simulink model "CAN_Model_v5"  (R2018b)
settings: Solver=VariableStepAuto  StartTime=0.0  StopTime=SimTime  RelTol=1e-3
InitFcn:
  | run('CAN_ModelMat.m')
values from neighbouring files (symbols this model uses):
  ID = [1,0,0,0,0,1,1,0,0,1,0]    [CAN_ModelMat.m]    (also in CAN_ModelMatv2.m = [1,1,1,1,1,0,0,1,1,1,1]; stuff.m = [ID(1:i) 0 ID(i+1:end)])
  NodesID = [ 0,0,1,1,0,1,1,0,0,1,1 ... (first row only)    [CAN_ModelMat.m]    (also in CAN_ModelMatv2.m)
  RandPayload = randi([0,1],1, 64)    [CAN_ModelMat.m]
  RTS_Inc = round(SimTime / CLK / NumOfFrames)    [CAN_ModelMat.m]    (also in CAN_ModelMatv2.m)
  time = NodeTiming / CLK    (= 5000)    [CAN_ModelMat.m]    (also in CAN_ModelMatv2.m)
libraries: simulink_extras x1
settings Model: Creator=Emiliano  LastModifiedBy=MAX_1

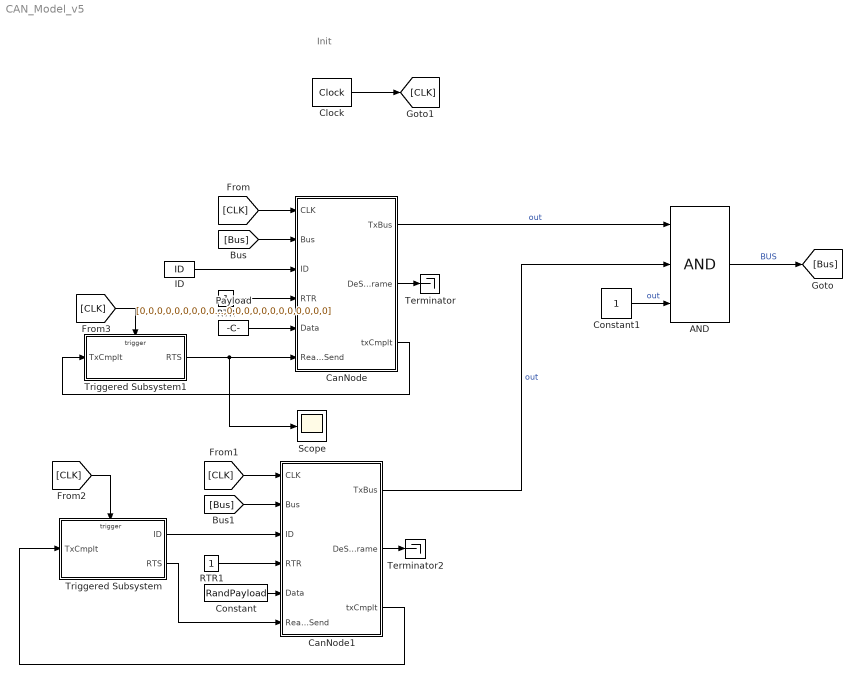
== system CAN_Model_v5 ==
  note: Init
  AND : Logic  Inputs=3  IconShape=distinctive  AllPortsSameDT=off  OutDataTypeStr=boolean
  CanNode : Subsystem
  CanNode1 : Subsystem
  Clock : simulink_extras/Flip Flops/Clock  period=CLK
  Constant : Constant  Value=RandPayload
  Constant1 : Constant
  ID : Constant  Value=ID
  "Payload " : Constant  Value=[0,0,0,0,0,0,0,0,0,0,0,0,0,0,0,0,0,0,0,0,0,0,0,0,0,0,0,0,0,0,0,0,0,0,0,0,0,0,0,0,0,0,0,0,0,0,0,0,0,0,0,0,0,0,0,0,0,0,0,0,0,0,0,0]
  RTR : Constant
  RTR1 : Constant
  Scope : Scope
  Terminator : Terminator
  Terminator2 : Terminator
  Triggered Subsystem : Subsystem  TreatAsAtomicUnit=on
  Triggered Subsystem1 : Subsystem  TreatAsAtomicUnit=on
  wires:
  CanNode/1("TxBus ") -> AND/1  "out"
  [Bus] -> CanNode/2(Bus)
  Triggered Subsystem1/1(RTS) -> Scope/1, CanNode/6("ReadyToSend ")
  ID/1 -> CanNode/3(ID)
  "Payload "/1 -> CanNode/5(Data)
  RTR/1 -> CanNode/4(RTR)
  Constant1/1 -> AND/3  "out"
  AND/1 -> [Bus]  "BUS"
  Clock/1 -> [CLK]
  [CLK] -> CanNode/1(CLK)
  CanNode/2(DeStuffedFrame) -> Terminator/1
  Triggered Subsystem/2(RTS) -> CanNode1/6("ReadyToSend ")
  [CLK] -> CanNode1/1(CLK)
  [Bus] -> CanNode1/2(Bus)
  CanNode1/1("TxBus ") -> AND/2  "out"
  CanNode1/3(txCmplt) -> Triggered Subsystem/1(TxCmplt)
  RTR1/1 -> CanNode1/4(RTR)
  CanNode1/2(DeStuffedFrame) -> Terminator2/1
  [CLK] -> Triggered Subsystem/Trigger
  Triggered Subsystem/1(ID) -> CanNode1/3(ID)
  [CLK] -> Triggered Subsystem1/Trigger
  CanNode/3(txCmplt) -> Triggered Subsystem1/1(TxCmplt)
  Constant/1 -> CanNode1/5(Data)

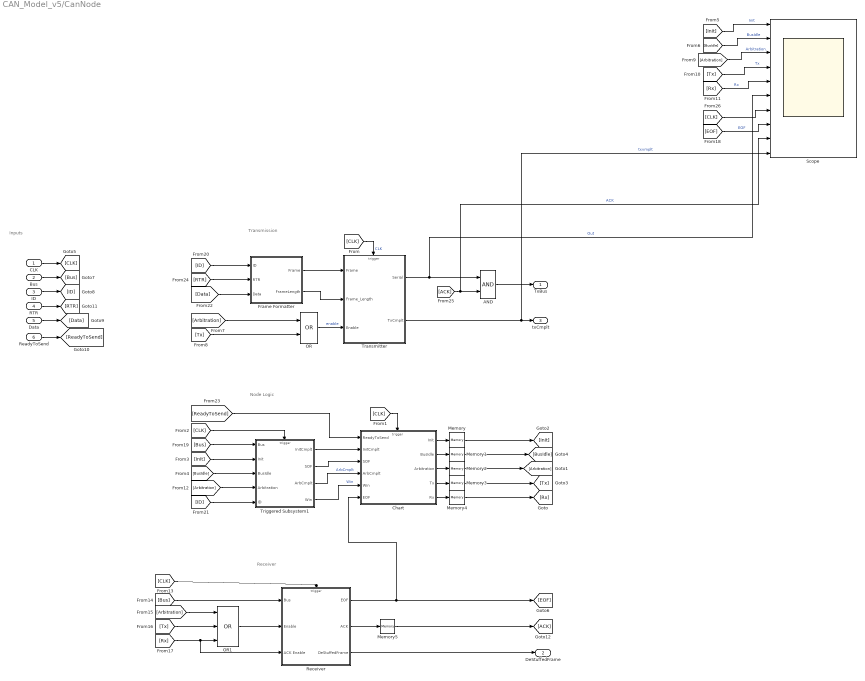
== system CAN_Model_v5/CanNode ==
  note: Transmission
  note: Node Logic
  note: Receiver
  note: Inputs
  CLK : Inport
  Bus : Inport  Port=2
  ID : Inport  Port=3
  RTR : Inport  Port=4
  Data : Inport  Port=5
  "ReadyToSend " : Inport  Port=6
  AND : Logic  IconShape=distinctive  AllPortsSameDT=off  OutDataTypeStr=boolean
  Chart : Stateflow chart  TreatAsAtomicUnit=on
  Frame Formatter : Subsystem
  Memory{,1..5} (6 alike) : Memory
  OR : Logic  Operator=OR  IconShape=distinctive  AllPortsSameDT=off  OutDataTypeStr=boolean
  OR1 : Logic  Operator=OR  Inputs=3  IconShape=distinctive  AllPortsSameDT=off  OutDataTypeStr=boolean
  Receiver : Subsystem  TreatAsAtomicUnit=on
  Scope : Scope  NumInputPorts=10
  Transmitter : Subsystem  TreatAsAtomicUnit=on
  Triggered Subsystem1 : Subsystem  TreatAsAtomicUnit=on
  "TxBus " : Outport
  DeStuffedFrame : Outport  Port=2
  txCmplt : Outport  Port=3
  wires:
  [CLK] -> Chart/Trigger
  [Arbitration] -> OR/1
  [Tx] -> OR/2
  OR/1 -> Transmitter/3(Enable)  "enable"
  Chart/5(" Rx") -> Memory4/1
  Chart/3(" Arbitration") -> Memory2/1
  Chart/1(" Init") -> Memory/1
  Chart/4(" Tx") -> Memory3/1
  Chart/2(" BusIdle") -> Memory1/1
  CLK/1 -> [CLK]
  [CLK] -> Transmitter/Trigger  "CLK"
  [CLK] -> Triggered Subsystem1/Trigger
  [Init] -> Triggered Subsystem1/2(Init)
  [BusIdle] -> Triggered Subsystem1/3(BusIdle)
  Triggered Subsystem1/2(SOF) -> Chart/3(SOF)
  Triggered Subsystem1/3("ArbCmplt ") -> Chart/4(ArbCmplt)  "ArbCmplt"
  [Init] -> Scope/1  "Init"
  [BusIdle] -> Scope/2  "BusIdle"
  [Arbitration] -> Scope/3  "Arbitration"
  [Tx] -> Scope/4  "Tx"
  [Rx] -> Scope/5  "Rx"
  Memory/1 -> [Init]
  Memory1/1 -> [BusIdle]
  Memory2/1 -> [Arbitration]
  Memory3/1 -> [Tx]
  Memory4/1 -> [Rx]
  Transmitter/1(Serial) -> Scope/6, AND/1  "Out"
  [Arbitration] -> Triggered Subsystem1/4(Arbitration)
  [CLK] -> Receiver/Trigger
  [Bus] -> Receiver/1(Bus)
  [Arbitration] -> OR1/1
  [Tx] -> OR1/2
  Receiver/1(EOF) -> Chart/6(EOF), [EOF]
  [EOF] -> Scope/8  "EOF"
  Bus/1 -> [Bus]
  [Bus] -> Triggered Subsystem1/1(Bus)
  Frame Formatter/1(Frame) -> Transmitter/1("Frame ")
  Frame Formatter/2("FrameLength ") -> Transmitter/2(Frame_Length)
  ID/1 -> [ID]
  [ID] -> Frame Formatter/1(ID)
  [ID] -> Triggered Subsystem1/5(ID)
  Data/1 -> [Data]
  "ReadyToSend "/1 -> [ReadyToSend]
  [ReadyToSend] -> Chart/1(ReadyToSend)
  [Data] -> Frame Formatter/3(Data)
  RTR/1 -> [RTR]
  [RTR] -> Frame Formatter/2(RTR)
  Receiver/2(ACK) -> Memory5/1
  Triggered Subsystem1/4(Win) -> Chart/5(Win)  "Win"
  Memory5/1 -> [ACK]
  AND/1 -> "TxBus "/1
  [ACK] -> Scope/9, AND/2  "ACK"
  Triggered Subsystem1/1(InitCmplt) -> Chart/2(InitCmplt)
  [CLK] -> Scope/7
  Receiver/3(DeStuffedFrame) -> DeStuffedFrame/1
  OR1/1 -> Receiver/2(Enable)
  [Rx] -> Receiver/3(ACK Enable), OR1/3
  Transmitter/2(TxCmplt) -> Scope/10, txCmplt/1  "txvmplt"

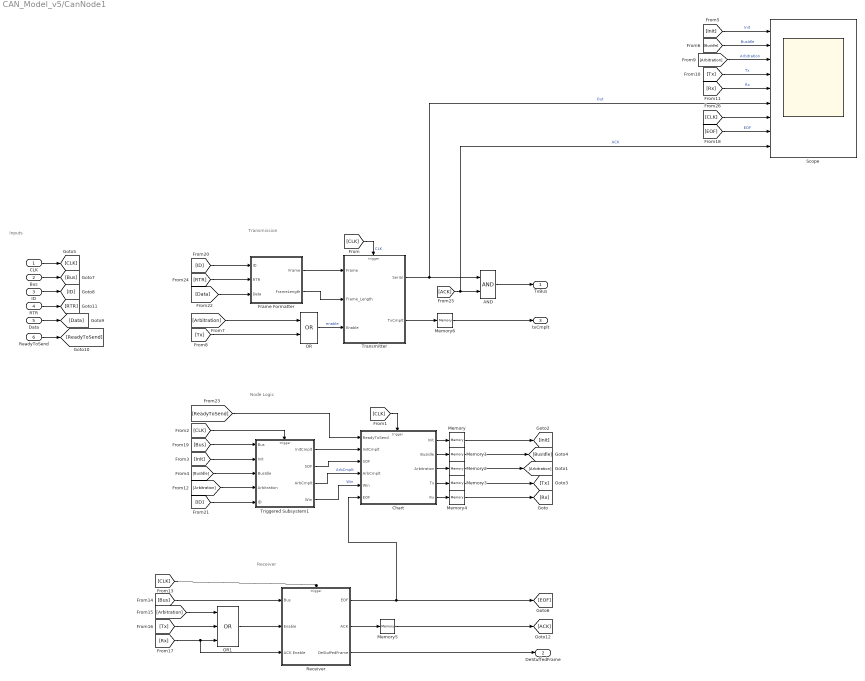
== system CAN_Model_v5/CanNode1 ==
  note: Transmission
  note: Node Logic
  note: Receiver
  note: Inputs
  CLK : Inport
  Bus : Inport  Port=2
  ID : Inport  Port=3
  RTR : Inport  Port=4
  Data : Inport  Port=5
  "ReadyToSend " : Inport  Port=6
  AND : Logic  IconShape=distinctive  AllPortsSameDT=off  OutDataTypeStr=boolean
  Chart : Stateflow chart  TreatAsAtomicUnit=on
  Frame Formatter : Subsystem
  Memory{,1..6} (7 alike) : Memory
  OR : Logic  Operator=OR  IconShape=distinctive  AllPortsSameDT=off  OutDataTypeStr=boolean
  OR1 : Logic  Operator=OR  Inputs=3  IconShape=distinctive  AllPortsSameDT=off  OutDataTypeStr=boolean
  Receiver : Subsystem  TreatAsAtomicUnit=on
  Scope : Scope  NumInputPorts=9
  Transmitter : Subsystem  TreatAsAtomicUnit=on
  Triggered Subsystem1 : Subsystem  TreatAsAtomicUnit=on
  "TxBus " : Outport
  DeStuffedFrame : Outport  Port=2
  txCmplt : Outport  Port=3
  wires:
  [CLK] -> Chart/Trigger
  [Arbitration] -> OR/1
  [Tx] -> OR/2
  OR/1 -> Transmitter/3(Enable)  "enable"
  Chart/5(" Rx") -> Memory4/1
  Chart/3(" Arbitration") -> Memory2/1
  Chart/1(" Init") -> Memory/1
  Chart/4(" Tx") -> Memory3/1
  Chart/2(" BusIdle") -> Memory1/1
  CLK/1 -> [CLK]
  [CLK] -> Transmitter/Trigger  "CLK"
  [CLK] -> Triggered Subsystem1/Trigger
  [Init] -> Triggered Subsystem1/2(Init)
  [BusIdle] -> Triggered Subsystem1/3(BusIdle)
  Triggered Subsystem1/2(SOF) -> Chart/3(SOF)
  Triggered Subsystem1/3("ArbCmplt ") -> Chart/4(ArbCmplt)  "ArbCmplt"
  [Init] -> Scope/1  "Init"
  [BusIdle] -> Scope/2  "BusIdle"
  [Arbitration] -> Scope/3  "Arbitration"
  [Tx] -> Scope/4  "Tx"
  [Rx] -> Scope/5  "Rx"
  Memory/1 -> [Init]
  Memory1/1 -> [BusIdle]
  Memory2/1 -> [Arbitration]
  Memory3/1 -> [Tx]
  Memory4/1 -> [Rx]
  Transmitter/1(Serial) -> Scope/6, AND/1  "Out"
  [Arbitration] -> Triggered Subsystem1/4(Arbitration)
  [CLK] -> Receiver/Trigger
  [Bus] -> Receiver/1(Bus)
  [Arbitration] -> OR1/1
  [Tx] -> OR1/2
  Receiver/1(EOF) -> Chart/6(EOF), [EOF]
  [EOF] -> Scope/8  "EOF"
  Bus/1 -> [Bus]
  [Bus] -> Triggered Subsystem1/1(Bus)
  Frame Formatter/1(Frame) -> Transmitter/1("Frame ")
  Frame Formatter/2("FrameLength ") -> Transmitter/2(Frame_Length)
  ID/1 -> [ID]
  [ID] -> Frame Formatter/1(ID)
  [ID] -> Triggered Subsystem1/5(ID)
  Data/1 -> [Data]
  "ReadyToSend "/1 -> [ReadyToSend]
  [ReadyToSend] -> Chart/1(ReadyToSend)
  [Data] -> Frame Formatter/3(Data)
  RTR/1 -> [RTR]
  [RTR] -> Frame Formatter/2(RTR)
  Receiver/2(ACK) -> Memory5/1
  Triggered Subsystem1/4(Win) -> Chart/5(Win)  "Win"
  Memory5/1 -> [ACK]
  AND/1 -> "TxBus "/1
  [ACK] -> Scope/9, AND/2  "ACK"
  Triggered Subsystem1/1(InitCmplt) -> Chart/2(InitCmplt)
  [CLK] -> Scope/7
  Receiver/3(DeStuffedFrame) -> DeStuffedFrame/1
  OR1/1 -> Receiver/2(Enable)
  [Rx] -> Receiver/3(ACK Enable), OR1/3
  Transmitter/2(TxCmplt) -> Memory6/1
  Memory6/1 -> txCmplt/1

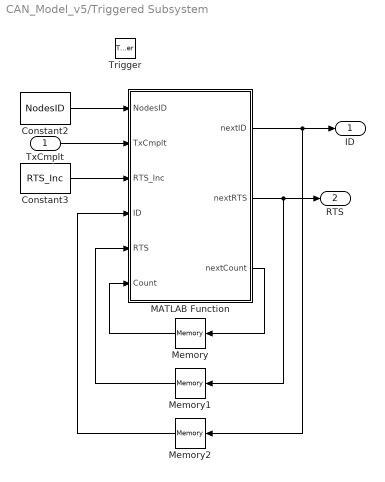
== system CAN_Model_v5/Triggered Subsystem ==
  TxCmplt : Inport
  Trigger : TriggerPort  VariantControl=Variant
  Constant2 : Constant  Value=NodesID
  Constant3 : Constant  Value=RTS_Inc
  MATLAB Function : MATLAB Function  TreatAsAtomicUnit=on
  Memory : Memory  InheritSampleTime=on
  Memory1 : Memory  InheritSampleTime=on
  Memory2 : Memory  InitialCondition=NodesID(1,:)  InheritSampleTime=on
  ID : Outport
  RTS : Outport  Port=2
  wires:
  Constant2/1 -> MATLAB Function/1(NodesID)
  MATLAB Function/3(nextCount) -> Memory/1
  Memory/1 -> MATLAB Function/6(Count)
  MATLAB Function/2(nextRTS) -> RTS/1, Memory1/1
  Memory1/1 -> MATLAB Function/5(RTS)
  MATLAB Function/1(nextID) -> ID/1, Memory2/1
  Memory2/1 -> MATLAB Function/4(ID)
  Constant3/1 -> MATLAB Function/3(RTS_Inc)
  TxCmplt/1 -> MATLAB Function/2(TxCmplt)

== system CAN_Model_v5/Triggered Subsystem1 ==
  TxCmplt : Inport
  Trigger : TriggerPort  VariantControl=Variant
  Constant : Constant  Value=time
  MATLAB Function : MATLAB Function  TreatAsAtomicUnit=on
  Memory : Memory  InheritSampleTime=on
  Memory1 : Memory  InheritSampleTime=on
  RTS : Outport
  wires:
  MATLAB Function/1(nextRTS) -> Memory1/1, RTS/1
  Constant/1 -> MATLAB Function/1(Timer)
  TxCmplt/1 -> MATLAB Function/2(TxCmplt)
  MATLAB Function/2(nextCount) -> Memory/1
  Memory/1 -> MATLAB Function/4(Count)
  Memory1/1 -> MATLAB Function/3(RTS)

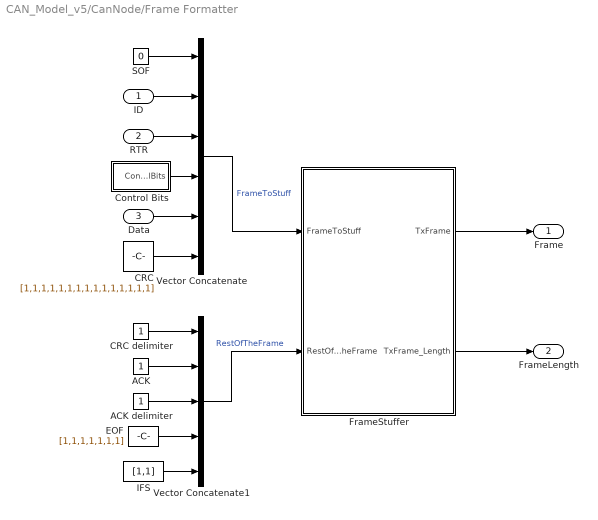
== system CAN_Model_v5/CanNode/Frame Formatter ==
  ID : Inport
  RTR : Inport  Port=2
  Data : Inport  Port=3
  ACK : Constant
  ACK delimiter : Constant
  CRC : Constant  Value=[1,1,1,1,1,1,1,1,1,1,1,1,1,1,1]
  CRC delimiter : Constant  VectorParams1D=off
  Control Bits : Subsystem
  EOF : Constant  Value=[1,1,1,1,1,1,1]
  FrameStuffer : Subsystem
  IFS : Constant  Value=[1,1]
  SOF : Constant  Value=0
  Vector Concatenate : Concatenate  NumInputs=6
  Vector Concatenate1 : Concatenate  NumInputs=5
  Frame : Outport
  "FrameLength " : Outport  Port=2
  wires:
  ID/1 -> Vector Concatenate/2
  RTR/1 -> Vector Concatenate/3
  Vector Concatenate/1 -> FrameStuffer/1(FrameToStuff)  "FrameToStuff"
  FrameStuffer/1(TxFrame) -> Frame/1
  FrameStuffer/2(TxFrame_Length) -> "FrameLength "/1
  SOF/1 -> Vector Concatenate/1
  Control Bits/1(ControlBits) -> Vector Concatenate/4
  Data/1 -> Vector Concatenate/5
  CRC/1 -> Vector Concatenate/6
  CRC delimiter/1 -> Vector Concatenate1/1
  ACK/1 -> Vector Concatenate1/2
  ACK delimiter/1 -> Vector Concatenate1/3
  EOF/1 -> Vector Concatenate1/4
  IFS/1 -> Vector Concatenate1/5
  Vector Concatenate1/1 -> FrameStuffer/2(RestOfTheFrame)  "RestOfTheFrame"

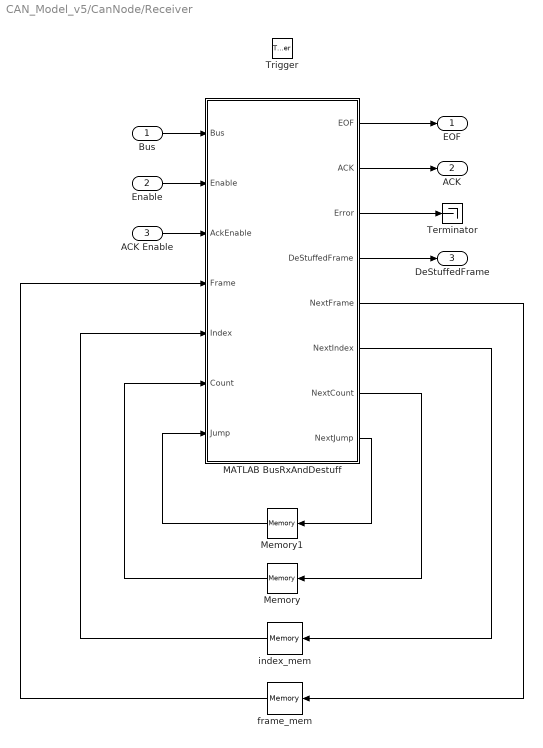
== system CAN_Model_v5/CanNode/Receiver ==
  Bus : Inport
  Enable : Inport  Port=2
  ACK Enable : Inport  Port=3
  Trigger : TriggerPort  VariantControl=Variant
  MATLAB BusRxAndDestuff : MATLAB Function  TreatAsAtomicUnit=on
  Memory : Memory  InheritSampleTime=on
  Memory1 : Memory  InheritSampleTime=on
  Terminator : Terminator
  frame_mem : Memory  InitialCondition=[0,0,0,0,0,0,0,0,0,0,0,0,0,0,0,0,0,0,0,0,0,0,0,0,0,0,0,0,0,0,0,0,0,0,0,0,0,0,0,0,0,0,0,0,0,0,0,0,0,0,0,0,0,0,0,0,0,0,0,0,0,0,0,0,0,0,0,0,0,0,0,0,0,0,0,0,0,0,0,0,0,0,0,0,0,0,0,0,0,0,0,0,0,0,0,0,0,0,0,0,0,0,0,0,0,0,0,0,0,0]  InheritSampleTime=on
  index_mem : Memory  InitialCondition=1  InheritSampleTime=on
  EOF : Outport
  ACK : Outport  Port=2
  DeStuffedFrame : Outport  Port=3
  wires:
  Enable/1 -> MATLAB BusRxAndDestuff/2(Enable)
  Bus/1 -> MATLAB BusRxAndDestuff/1(Bus)
  MATLAB BusRxAndDestuff/6(NextIndex) -> index_mem/1
  frame_mem/1 -> MATLAB BusRxAndDestuff/4(Frame)
  MATLAB BusRxAndDestuff/1(EOF) -> EOF/1
  MATLAB BusRxAndDestuff/5(NextFrame) -> frame_mem/1
  index_mem/1 -> MATLAB BusRxAndDestuff/5(Index)
  MATLAB BusRxAndDestuff/3(Error) -> Terminator/1
  MATLAB BusRxAndDestuff/7(NextCount) -> Memory/1
  Memory/1 -> MATLAB BusRxAndDestuff/6(Count)
  MATLAB BusRxAndDestuff/8(NextJump) -> Memory1/1
  Memory1/1 -> MATLAB BusRxAndDestuff/7(Jump)
  MATLAB BusRxAndDestuff/4(DeStuffedFrame) -> DeStuffedFrame/1
  MATLAB BusRxAndDestuff/2(ACK) -> ACK/1
  ACK Enable/1 -> MATLAB BusRxAndDestuff/3(AckEnable)

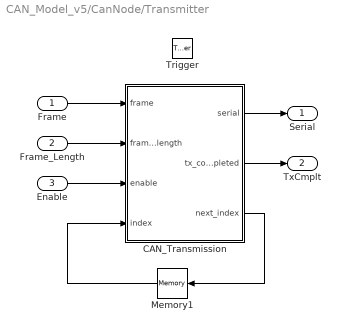
== system CAN_Model_v5/CanNode/Transmitter ==
  "Frame " : Inport
  Frame_Length : Inport  Port=2
  Enable : Inport  Port=3
  Trigger : TriggerPort  VariantControl=Variant
  CAN_Transmission : MATLAB Function  TreatAsAtomicUnit=on
  Memory1 : Memory  InitialCondition=1  InheritSampleTime=on
  Serial : Outport
  TxCmplt : Outport  Port=2
  wires:
  Memory1/1 -> CAN_Transmission/4(index)
  CAN_Transmission/1(serial) -> Serial/1
  CAN_Transmission/3(next_index) -> Memory1/1
  CAN_Transmission/2(tx_completed) -> TxCmplt/1
  Enable/1 -> CAN_Transmission/3(enable)
  "Frame "/1 -> CAN_Transmission/1(frame)
  Frame_Length/1 -> CAN_Transmission/2(frame_length)

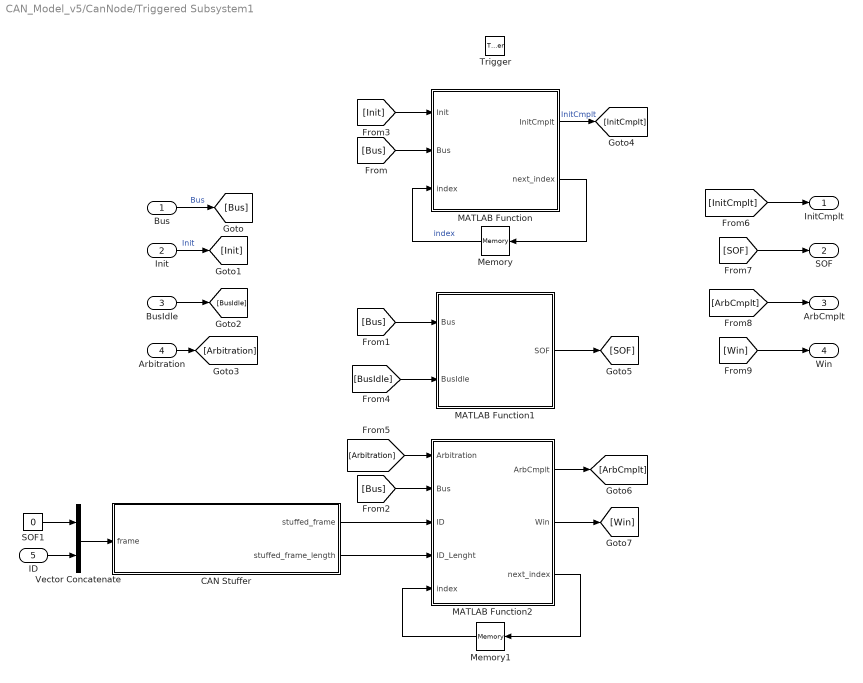
== system CAN_Model_v5/CanNode/Triggered Subsystem1 ==
  Bus : Inport
  Init : Inport  Port=2
  BusIdle : Inport  Port=3
  Arbitration : Inport  Port=4
  ID : Inport  Port=5
  Trigger : TriggerPort  VariantControl=Variant
  CAN Stuffer : MATLAB Function  TreatAsAtomicUnit=on
  MATLAB Function : MATLAB Function  TreatAsAtomicUnit=on
  MATLAB Function1 : MATLAB Function  TreatAsAtomicUnit=on
  MATLAB Function2 : MATLAB Function  TreatAsAtomicUnit=on
  Memory : Memory  InheritSampleTime=on
  Memory1 : Memory  InitialCondition=1  InheritSampleTime=on
  SOF1 : Constant  Value=0
  Vector Concatenate : Concatenate
  InitCmplt : Outport
  SOF : Outport  Port=2
  "ArbCmplt " : Outport  Port=3
  Win : Outport  Port=4
  wires:
  MATLAB Function/2(next_index) -> Memory/1
  Memory/1 -> MATLAB Function/3(index)  "index"
  Bus/1 -> [Bus]  "Bus"
  [Bus] -> MATLAB Function/2(Bus)
  [Bus] -> MATLAB Function1/1(Bus)
  [Bus] -> MATLAB Function2/2(Bus)
  MATLAB Function2/3(next_index) -> Memory1/1
  Memory1/1 -> MATLAB Function2/5(index)
  CAN Stuffer/1(stuffed_frame) -> MATLAB Function2/3(ID)
  CAN Stuffer/2(stuffed_frame_length) -> MATLAB Function2/4(ID_Lenght)
  SOF1/1 -> Vector Concatenate/1
  ID/1 -> Vector Concatenate/2
  Vector Concatenate/1 -> CAN Stuffer/1(frame)
  Init/1 -> [Init]  "Init"
  [Init] -> MATLAB Function/1(Init)
  BusIdle/1 -> [BusIdle]
  [BusIdle] -> MATLAB Function1/2(BusIdle)
  Arbitration/1 -> [Arbitration]
  [Arbitration] -> MATLAB Function2/1(Arbitration)
  MATLAB Function/1(InitCmplt) -> [InitCmplt]  "InitCmplt"
  [InitCmplt] -> InitCmplt/1
  MATLAB Function1/1(SOF) -> [SOF]
  [SOF] -> SOF/1
  MATLAB Function2/1(ArbCmplt) -> [ArbCmplt]
  [ArbCmplt] -> "ArbCmplt "/1
  [Win] -> Win/1
  MATLAB Function2/2(Win) -> [Win]

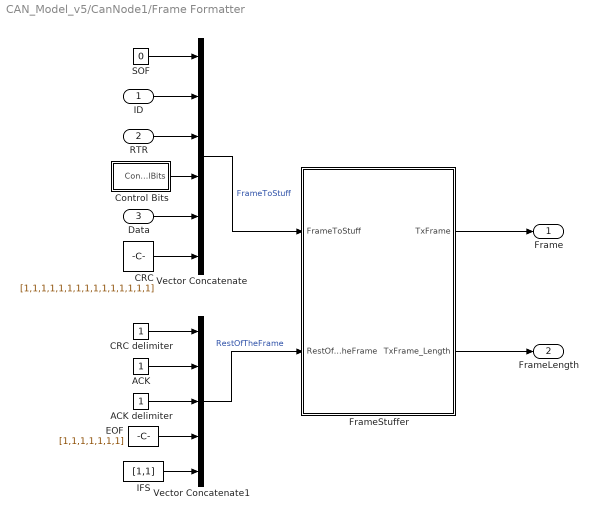
== system CAN_Model_v5/CanNode1/Frame Formatter ==
  ID : Inport
  RTR : Inport  Port=2
  Data : Inport  Port=3
  ACK : Constant
  ACK delimiter : Constant
  CRC : Constant  Value=[1,1,1,1,1,1,1,1,1,1,1,1,1,1,1]
  CRC delimiter : Constant  VectorParams1D=off
  Control Bits : Subsystem
  EOF : Constant  Value=[1,1,1,1,1,1,1]
  FrameStuffer : Subsystem
  IFS : Constant  Value=[1,1]
  SOF : Constant  Value=0
  Vector Concatenate : Concatenate  NumInputs=6
  Vector Concatenate1 : Concatenate  NumInputs=5
  Frame : Outport
  "FrameLength " : Outport  Port=2
  wires:
  ID/1 -> Vector Concatenate/2
  RTR/1 -> Vector Concatenate/3
  Vector Concatenate/1 -> FrameStuffer/1(FrameToStuff)  "FrameToStuff"
  FrameStuffer/1(TxFrame) -> Frame/1
  FrameStuffer/2(TxFrame_Length) -> "FrameLength "/1
  SOF/1 -> Vector Concatenate/1
  Control Bits/1(ControlBits) -> Vector Concatenate/4
  Data/1 -> Vector Concatenate/5
  CRC/1 -> Vector Concatenate/6
  CRC delimiter/1 -> Vector Concatenate1/1
  ACK/1 -> Vector Concatenate1/2
  ACK delimiter/1 -> Vector Concatenate1/3
  EOF/1 -> Vector Concatenate1/4
  IFS/1 -> Vector Concatenate1/5
  Vector Concatenate1/1 -> FrameStuffer/2(RestOfTheFrame)  "RestOfTheFrame"

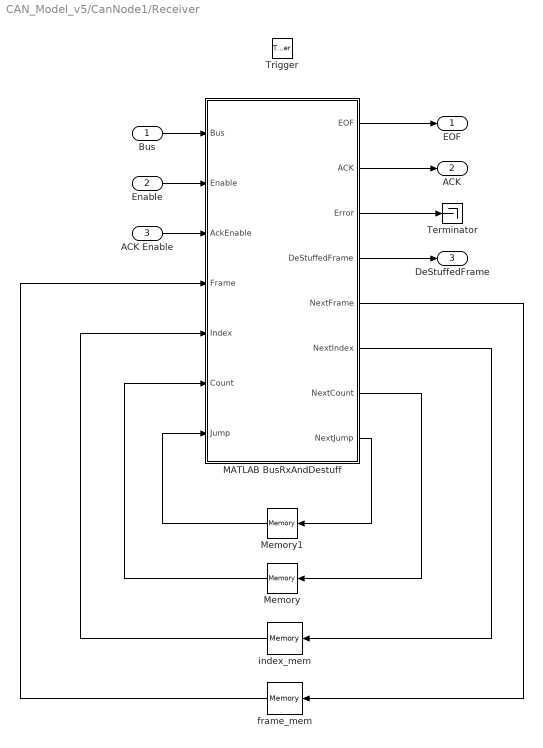
== system CAN_Model_v5/CanNode1/Receiver ==
  Bus : Inport
  Enable : Inport  Port=2
  ACK Enable : Inport  Port=3
  Trigger : TriggerPort  VariantControl=Variant
  MATLAB BusRxAndDestuff : MATLAB Function  TreatAsAtomicUnit=on
  Memory : Memory  InheritSampleTime=on
  Memory1 : Memory  InheritSampleTime=on
  Terminator : Terminator
  frame_mem : Memory  InitialCondition=[0,0,0,0,0,0,0,0,0,0,0,0,0,0,0,0,0,0,0,0,0,0,0,0,0,0,0,0,0,0,0,0,0,0,0,0,0,0,0,0,0,0,0,0,0,0,0,0,0,0,0,0,0,0,0,0,0,0,0,0,0,0,0,0,0,0,0,0,0,0,0,0,0,0,0,0,0,0,0,0,0,0,0,0,0,0,0,0,0,0,0,0,0,0,0,0,0,0,0,0,0,0,0,0,0,0,0,0,0,0]  InheritSampleTime=on
  index_mem : Memory  InitialCondition=1  InheritSampleTime=on
  EOF : Outport
  ACK : Outport  Port=2
  DeStuffedFrame : Outport  Port=3
  wires:
  Enable/1 -> MATLAB BusRxAndDestuff/2(Enable)
  Bus/1 -> MATLAB BusRxAndDestuff/1(Bus)
  MATLAB BusRxAndDestuff/6(NextIndex) -> index_mem/1
  frame_mem/1 -> MATLAB BusRxAndDestuff/4(Frame)
  MATLAB BusRxAndDestuff/1(EOF) -> EOF/1
  MATLAB BusRxAndDestuff/5(NextFrame) -> frame_mem/1
  index_mem/1 -> MATLAB BusRxAndDestuff/5(Index)
  MATLAB BusRxAndDestuff/3(Error) -> Terminator/1
  MATLAB BusRxAndDestuff/7(NextCount) -> Memory/1
  Memory/1 -> MATLAB BusRxAndDestuff/6(Count)
  MATLAB BusRxAndDestuff/8(NextJump) -> Memory1/1
  Memory1/1 -> MATLAB BusRxAndDestuff/7(Jump)
  MATLAB BusRxAndDestuff/4(DeStuffedFrame) -> DeStuffedFrame/1
  MATLAB BusRxAndDestuff/2(ACK) -> ACK/1
  ACK Enable/1 -> MATLAB BusRxAndDestuff/3(AckEnable)

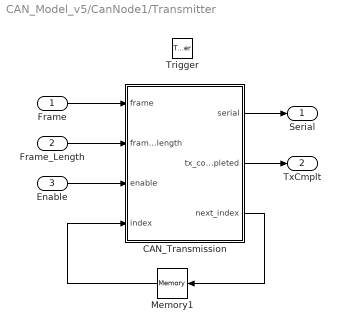
== system CAN_Model_v5/CanNode1/Transmitter ==
  "Frame " : Inport
  Frame_Length : Inport  Port=2
  Enable : Inport  Port=3
  Trigger : TriggerPort  VariantControl=Variant
  CAN_Transmission : MATLAB Function  TreatAsAtomicUnit=on
  Memory1 : Memory  InitialCondition=1  InheritSampleTime=on
  Serial : Outport
  TxCmplt : Outport  Port=2
  wires:
  Memory1/1 -> CAN_Transmission/4(index)
  CAN_Transmission/1(serial) -> Serial/1
  CAN_Transmission/3(next_index) -> Memory1/1
  CAN_Transmission/2(tx_completed) -> TxCmplt/1
  Enable/1 -> CAN_Transmission/3(enable)
  "Frame "/1 -> CAN_Transmission/1(frame)
  Frame_Length/1 -> CAN_Transmission/2(frame_length)

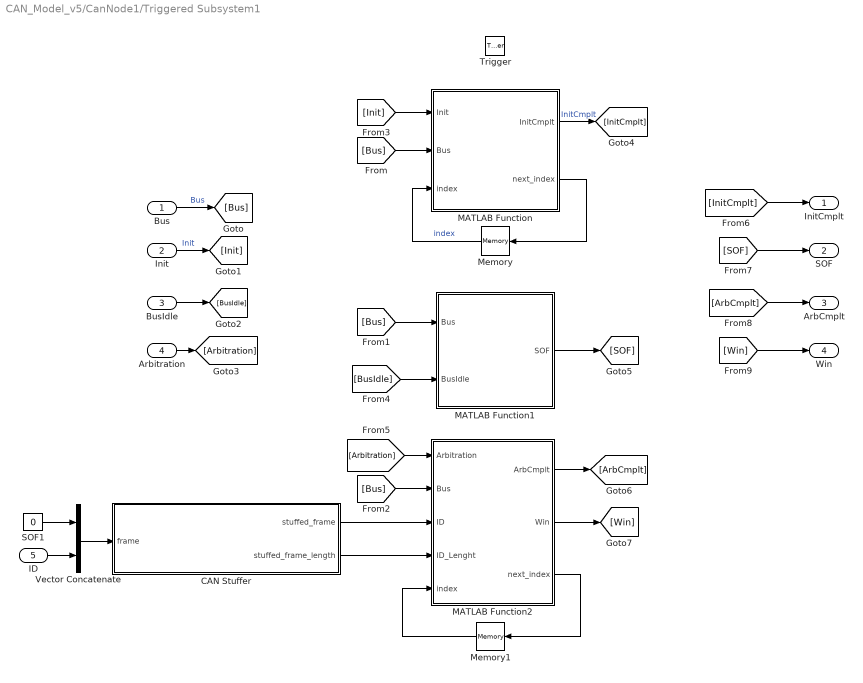
== system CAN_Model_v5/CanNode1/Triggered Subsystem1 ==
  Bus : Inport
  Init : Inport  Port=2
  BusIdle : Inport  Port=3
  Arbitration : Inport  Port=4
  ID : Inport  Port=5
  Trigger : TriggerPort  VariantControl=Variant
  CAN Stuffer : MATLAB Function  TreatAsAtomicUnit=on
  MATLAB Function : MATLAB Function  TreatAsAtomicUnit=on
  MATLAB Function1 : MATLAB Function  TreatAsAtomicUnit=on
  MATLAB Function2 : MATLAB Function  TreatAsAtomicUnit=on
  Memory : Memory  InheritSampleTime=on
  Memory1 : Memory  InitialCondition=1  InheritSampleTime=on
  SOF1 : Constant  Value=0
  Vector Concatenate : Concatenate
  InitCmplt : Outport
  SOF : Outport  Port=2
  "ArbCmplt " : Outport  Port=3
  Win : Outport  Port=4
  wires:
  MATLAB Function/2(next_index) -> Memory/1
  Memory/1 -> MATLAB Function/3(index)  "index"
  Bus/1 -> [Bus]  "Bus"
  [Bus] -> MATLAB Function/2(Bus)
  [Bus] -> MATLAB Function1/1(Bus)
  [Bus] -> MATLAB Function2/2(Bus)
  MATLAB Function2/3(next_index) -> Memory1/1
  Memory1/1 -> MATLAB Function2/5(index)
  CAN Stuffer/1(stuffed_frame) -> MATLAB Function2/3(ID)
  CAN Stuffer/2(stuffed_frame_length) -> MATLAB Function2/4(ID_Lenght)
  SOF1/1 -> Vector Concatenate/1
  ID/1 -> Vector Concatenate/2
  Vector Concatenate/1 -> CAN Stuffer/1(frame)
  Init/1 -> [Init]  "Init"
  [Init] -> MATLAB Function/1(Init)
  BusIdle/1 -> [BusIdle]
  [BusIdle] -> MATLAB Function1/2(BusIdle)
  Arbitration/1 -> [Arbitration]
  [Arbitration] -> MATLAB Function2/1(Arbitration)
  MATLAB Function/1(InitCmplt) -> [InitCmplt]  "InitCmplt"
  [InitCmplt] -> InitCmplt/1
  MATLAB Function1/1(SOF) -> [SOF]
  [SOF] -> SOF/1
  MATLAB Function2/1(ArbCmplt) -> [ArbCmplt]
  [ArbCmplt] -> "ArbCmplt "/1
  [Win] -> Win/1
  MATLAB Function2/2(Win) -> [Win]

== system CAN_Model_v5/CanNode/Frame Formatter/Control Bits ==
  Control Bits : Concatenate  NumInputs=3
  DLC : Constant  Value=[1,0,0,0]
  IDE : Constant  Value=0
  Reserved : Constant  Value=0
  ControlBits : Outport
  wires:
  DLC/1 -> Control Bits/3
  IDE/1 -> Control Bits/1
  Reserved/1 -> Control Bits/2
  Control Bits/1 -> ControlBits/1

== system CAN_Model_v5/CanNode/Frame Formatter/FrameStuffer ==
  FrameToStuff : Inport
  RestOfTheFrame : Inport  Port=2
  CAN Stuffer : MATLAB Function  TreatAsAtomicUnit=on
  MATLAB Function : MATLAB Function  TreatAsAtomicUnit=on
  VectorLength : MATLAB Function  TreatAsAtomicUnit=on
  TxFrame : Outport
  TxFrame_Length : Outport  Port=2
  wires:
  MATLAB Function/2(LEN_C) -> TxFrame_Length/1
  MATLAB Function/1(C) -> TxFrame/1
  RestOfTheFrame/1 -> VectorLength/1(Vector), MATLAB Function/3(B)
  VectorLength/1(Length) -> MATLAB Function/4(LEN_B)
  FrameToStuff/1 -> CAN Stuffer/1(frame)
  CAN Stuffer/1(stuffed_frame) -> MATLAB Function/1(A)
  CAN Stuffer/2(stuffed_frame_length) -> MATLAB Function/2(LEN_A)

== system CAN_Model_v5/CanNode1/Frame Formatter/Control Bits ==
  Control Bits : Concatenate  NumInputs=3
  DLC : Constant  Value=[1,0,0,0]
  IDE : Constant  Value=0
  Reserved : Constant  Value=0
  ControlBits : Outport
  wires:
  DLC/1 -> Control Bits/3
  IDE/1 -> Control Bits/1
  Reserved/1 -> Control Bits/2
  Control Bits/1 -> ControlBits/1

== system CAN_Model_v5/CanNode1/Frame Formatter/FrameStuffer ==
  FrameToStuff : Inport
  RestOfTheFrame : Inport  Port=2
  CAN Stuffer : MATLAB Function  TreatAsAtomicUnit=on
  MATLAB Function : MATLAB Function  TreatAsAtomicUnit=on
  VectorLength : MATLAB Function  TreatAsAtomicUnit=on
  TxFrame : Outport
  TxFrame_Length : Outport  Port=2
  wires:
  MATLAB Function/2(LEN_C) -> TxFrame_Length/1
  MATLAB Function/1(C) -> TxFrame/1
  RestOfTheFrame/1 -> VectorLength/1(Vector), MATLAB Function/3(B)
  VectorLength/1(Length) -> MATLAB Function/4(LEN_B)
  FrameToStuff/1 -> CAN Stuffer/1(frame)
  CAN Stuffer/1(stuffed_frame) -> MATLAB Function/1(A)
  CAN Stuffer/2(stuffed_frame_length) -> MATLAB Function/2(LEN_A)

== matlab function CAN_Model_v5/CanNode/Triggered Subsystem1/MATLAB Function ==
  data: Init input; InitCmplt output; Bus input; index input; next_index output
function [InitCmplt, next_index] = BusIdleSensing(Init, Bus, index)

InitCmplt = 0;

if Init == 1
    if Bus == 1
        if index < 10 %Number of one to wait for EOF (after 11 ones)
            next_index = index + 1;
        else
            next_index = 0;
            InitCmplt = 1;
        end
    else
        next_index = 0;
    end
else
   next_index = 0;
end

end

== matlab function CAN_Model_v5/CanNode/Transmitter/CAN_Transmission ==
  data: frame input; frame_length input; enable input; serial output; tx_completed output; index input; next_index output
function [serial,  tx_completed ,next_index]  = fcn(frame, frame_length, enable, index)

if enable == 1
    if index == frame_length
        serial = frame(index);
        tx_completed = 1;
        next_index = 1;
    else
        serial = frame(index);
        next_index = index + 1;
        tx_completed = 0;
    end
else
    tx_completed = 0;
    serial = 1;
    next_index = 1;
end

end

== stateflow chart CAN_Model_v5/CanNode/Chart ==
  settings: sampleTime=0.2  executeAtInitialization=1
  state Init
  state Rx
  state BusIdle
  state Arbitration
  state Tx
  Init -> Init [order 2] : [InitCmplt == 0]
  (default) -> Init
  Init -> BusIdle [order 1] : [InitCmplt == 1]
  Rx -> Rx [order 2] : [EOF == 0]
  BusIdle -> Rx [order 2] : [ReadyToSend == 0 && SOF == 1]
  Rx -> BusIdle [order 1] : [EOF == 1]
  BusIdle -> BusIdle [order 3] : [ReadyToSend == 0 && SOF == 0]
  Arbitration -> Rx [order 1] : [ArbCmplt ==1 && Win == 0]
  Tx -> BusIdle [order 2] : [EOF == 1]
  BusIdle -> Arbitration [order 1] : [ReadyToSend > 0]
  Arbitration -> Tx [order 2] : [ArbCmplt ==1 && Win == 1]
  Arbitration -> Arbitration [order 3] : [ArbCmplt == 0]
  Tx -> Tx [order 1] : [EOF == 0]
  data: Init output boolean; BusIdle output boolean; Arbitration output boolean; Tx output boolean; Rx output boolean; ReadyToSend input; InitCmplt input; SOF input; ArbCmplt input; Win input; EOF input
  events: Start input FALLING_EDGE_EVENT

== matlab function CAN_Model_v5/CanNode/Triggered Subsystem1/MATLAB Function1 ==
  data: Bus input; SOF output; BusIdle input
function SOF = SOF_Detection(Bus, BusIdle)

if BusIdle == 1 %Checks the current state of the FSM
    if Bus == 0
        SOF = 1; %SOF Detected, the flag goes to One!
    else
        SOF = 0;    
    end
else
    SOF = 0;
end

end

== matlab function CAN_Model_v5/CanNode/Triggered Subsystem1/MATLAB Function2 ==
  data: ArbCmplt output; Win output; Arbitration input; Bus input; ID input; ID_Lenght input; next_index output; index input
function [ArbCmplt, Win, next_index] = arbitration(Arbitration, Bus, ID, ID_Lenght, index)

ArbCmplt = 0;
Win = 0;
next_index = 1;

if Arbitration == 1
    if index <= ID_Lenght
        if ID(index) == Bus
            next_index = index + 1;
        else
            Win = 0;
            ArbCmplt = 1;
        end
    else
        next_index = 1;
        Win = 1;
        ArbCmplt = 1;
    end    
    
else next_index = 1;
    
end
end

== matlab function CAN_Model_v5/CanNode/Triggered Subsystem1/CAN Stuffer ==
  data: frame input; stuffed_frame output; stuffed_frame_length output
function [stuffed_frame, stuffed_frame_length] = CANstuffer(frame)

NumOfZeros = 0;
NumOfOnes = 0;
NumOfStuffedBits = 0;

stuffed_frame = zeros(135,1);

for i = 1 : length(frame)
    if frame(i) == 0
        NumOfZeros = NumOfZeros + 1;
        NumOfOnes = 0;
    else
        NumOfOnes = NumOfOnes + 1;
        NumOfZeros = 0;
    end
    
    if NumOfZeros == 5
        NumOfZeros = 0;
        NumOfOnes = NumOfOnes + 1;
        
        %Appending the stuffed ONE
        stuffed_frame(i + NumOfStuffedBits) = frame(i);
        NumOfStuffedBits = NumOfStuffedBits + 1;
        stuffed_frame(i + NumOfStuffedBits) = 1;
        
    elseif NumOfOnes == 5
        NumOfOnes = 0;
        NumOfZeros = NumOfZeros + 1;
        
        %Appending the stuffed ZERO
        stuffed_frame(i + NumOfStuffedBits) = frame(i);
        NumOfStuffedBits = NumOfStuffedBits + 1;
        stuffed_frame(i + NumOfStuffedBits) = 0;
        
    else
        stuffed_frame(i + NumOfStuffedBits) = frame(i); 
    end
end
stuffed_frame_length = length(frame) + NumOfStuffedBits;
end

== stateflow chart CAN_Model_v5/CanNode1/Chart ==
  settings: sampleTime=0.2  executeAtInitialization=1
  state Init
  state Rx
  state BusIdle
  state Arbitration
  state Tx
  Init -> Init [order 2] : [InitCmplt == 0]
  (default) -> Init
  Init -> BusIdle [order 1] : [InitCmplt == 1]
  Rx -> Rx [order 2] : [EOF == 0]
  BusIdle -> Rx [order 2] : [ReadyToSend == 0 && SOF == 1]
  Rx -> BusIdle [order 1] : [EOF == 1]
  BusIdle -> BusIdle [order 3] : [ReadyToSend == 0 && SOF == 0]
  Arbitration -> Rx [order 1] : [ArbCmplt ==1 && Win == 0]
  Tx -> BusIdle [order 2] : [EOF == 1]
  BusIdle -> Arbitration [order 1] : [ReadyToSend > 0]
  Arbitration -> Tx [order 2] : [ArbCmplt ==1 && Win == 1]
  Arbitration -> Arbitration [order 3] : [ArbCmplt == 0]
  Tx -> Tx [order 1] : [EOF == 0]
  data: Init output boolean; BusIdle output boolean; Arbitration output boolean; Tx output boolean; Rx output boolean; ReadyToSend input; InitCmplt input; SOF input; ArbCmplt input; Win input; EOF input
  events: Start input FALLING_EDGE_EVENT

== matlab function CAN_Model_v5/CanNode/Frame Formatter/FrameStuffer/CAN Stuffer ==
  data: stuffed_frame output; stuffed_frame_length output; frame input
function [stuffed_frame, stuffed_frame_length] = CANstuffer(frame)

NumOfZeros = 0;
NumOfOnes = 0;
NumOfStuffedBits = 0;

stuffed_frame = zeros(135,1);

for i = 1 : length(frame)
    if frame(i) == 0
        NumOfZeros = NumOfZeros + 1;
        NumOfOnes = 0;
    else
        NumOfOnes = NumOfOnes + 1;
        NumOfZeros = 0;
    end
    
    if NumOfZeros == 5
        NumOfZeros = 0;
        NumOfOnes = NumOfOnes + 1;
        
        %Appending the stuffed ONE
        stuffed_frame(i + NumOfStuffedBits) = frame(i);
        NumOfStuffedBits = NumOfStuffedBits + 1;
        stuffed_frame(i + NumOfStuffedBits) = 1;
        
    elseif NumOfOnes == 5
        NumOfOnes = 0;
        NumOfZeros = NumOfZeros + 1;
        
        %Appending the stuffed ZERO
        stuffed_frame(i + NumOfStuffedBits) = frame(i);
        NumOfStuffedBits = NumOfStuffedBits + 1;
        stuffed_frame(i + NumOfStuffedBits) = 0;
        
    else
        stuffed_frame(i + NumOfStuffedBits) = frame(i); 
    end
end
stuffed_frame_length = length(frame) + NumOfStuffedBits;
end

== matlab function CAN_Model_v5/CanNode/Frame Formatter/FrameStuffer/MATLAB Function ==
  data: A input; C output; LEN_A input; B input; LEN_B input; LEN_C output
function [C, LEN_C] = vectorAppend(A, LEN_A, B, LEN_B)

C = zeros(135,1);

for i = 1 : LEN_A
    C(i) = A(i);
end

for i = 1 : LEN_B
    C(LEN_A + i) = B(i);
end

LEN_C = LEN_A + LEN_B;
end

== matlab function CAN_Model_v5/CanNode/Frame Formatter/FrameStuffer/VectorLength ==
  data: Vector input; Length output
function Length = VectorLength(Vector)
Length = length(Vector);
end

== matlab function CAN_Model_v5/CanNode1/Frame Formatter/FrameStuffer/CAN Stuffer ==
  data: stuffed_frame output; stuffed_frame_length output; frame input
function [stuffed_frame, stuffed_frame_length] = CANstuffer(frame)

NumOfZeros = 0;
NumOfOnes = 0;
NumOfStuffedBits = 0;

stuffed_frame = zeros(135,1);

for i = 1 : length(frame)
    if frame(i) == 0
        NumOfZeros = NumOfZeros + 1;
        NumOfOnes = 0;
    else
        NumOfOnes = NumOfOnes + 1;
        NumOfZeros = 0;
    end
    
    if NumOfZeros == 5
        NumOfZeros = 0;
        NumOfOnes = NumOfOnes + 1;
        
        %Appending the stuffed ONE
        stuffed_frame(i + NumOfStuffedBits) = frame(i);
        NumOfStuffedBits = NumOfStuffedBits + 1;
        stuffed_frame(i + NumOfStuffedBits) = 1;
        
    elseif NumOfOnes == 5
        NumOfOnes = 0;
        NumOfZeros = NumOfZeros + 1;
        
        %Appending the stuffed ZERO
        stuffed_frame(i + NumOfStuffedBits) = frame(i);
        NumOfStuffedBits = NumOfStuffedBits + 1;
        stuffed_frame(i + NumOfStuffedBits) = 0;
        
    else
        stuffed_frame(i + NumOfStuffedBits) = frame(i); 
    end
end
stuffed_frame_length = length(frame) + NumOfStuffedBits;
end

== matlab function CAN_Model_v5/CanNode1/Frame Formatter/FrameStuffer/MATLAB Function ==
  data: A input; C output; LEN_A input; B input; LEN_B input; LEN_C output
function [C, LEN_C] = vectorAppend(A, LEN_A, B, LEN_B)

C = zeros(135,1);

for i = 1 : LEN_A
    C(i) = A(i);
end

for i = 1 : LEN_B
    C(LEN_A + i) = B(i);
end

LEN_C = LEN_A + LEN_B;
end

== matlab function CAN_Model_v5/CanNode1/Frame Formatter/FrameStuffer/VectorLength ==
  data: Vector input; Length output
function Length = VectorLength(Vector)
Length = length(Vector);
end

== matlab function CAN_Model_v5/CanNode1/Receiver/MATLAB BusRxAndDestuff ==
  data: Bus input; EOF output; ACK output; Enable input; AckEnable input; Frame input; Index input; Error output; DeStuffedFrame output; NextFrame output; NextIndex output; Count input; NextCount output; Jump input; NextJump output
function [EOF, ACK, Error, DeStuffedFrame, NextFrame, NextIndex, NextCount, NextJump] = BusRxAndDestuff(Bus, Enable, AckEnable, Frame, Index, Count, Jump)

DeStuffedFrame = zeros(110,1);
NextCount = 0;
NextFrame = zeros(110,1);
EOF = 0;
Error = 0;
NextIndex = 1;
NextJump = 0;
ACK = 1;

if Enable == 1
    if Index <= 110
        NextFrame = Frame;
        if (Index <= 98) || (Count == 4)
            if (Index == 1) || (Jump == 1)
                NextFrame(Index) = Bus;
                NextIndex = Index + 1;
            else
                if Count == 4
                    NextIndex = Index;
                    NextCount = 0;
                    NextJump = 1;
                else
                    NextFrame(Index) = Bus;
                    NextIndex = Index + 1;
                    if Bus == NextFrame(Index - 1)
                        NextCount = Count + 1;
                    else
                        NextCount = 0;
                    end
                end
            end
        else
            if(Index == 99) && (AckEnable == 1)
                ACK = 0;
            end
            NextFrame(Index) = Bus;
            NextIndex = Index + 1;
        end
    else
        EOF = 1;
        DeStuffedFrame = Frame;
    end
end
end

== matlab function CAN_Model_v5/CanNode1/Transmitter/CAN_Transmission ==
  data: frame input; frame_length input; enable input; serial output; tx_completed output; index input; next_index output
function [serial,  tx_completed ,next_index]  = fcn(frame, frame_length, enable, index)

if enable == 1
    if index == frame_length
        serial = frame(index);
        tx_completed = 1;
        next_index = 1;
    else
        serial = frame(index);
        next_index = index + 1;
        tx_completed = 0;
    end
else
    tx_completed = 0;
    serial = 1;
    next_index = 1;
end

end

== matlab function CAN_Model_v5/CanNode1/Triggered Subsystem1/CAN Stuffer ==
  data: frame input; stuffed_frame output; stuffed_frame_length output
function [stuffed_frame, stuffed_frame_length] = CANstuffer(frame)

NumOfZeros = 0;
NumOfOnes = 0;
NumOfStuffedBits = 0;

stuffed_frame = zeros(135,1);

for i = 1 : length(frame)
    if frame(i) == 0
        NumOfZeros = NumOfZeros + 1;
        NumOfOnes = 0;
    else
        NumOfOnes = NumOfOnes + 1;
        NumOfZeros = 0;
    end
    
    if NumOfZeros == 5
        NumOfZeros = 0;
        NumOfOnes = NumOfOnes + 1;
        
        %Appending the stuffed ONE
        stuffed_frame(i + NumOfStuffedBits) = frame(i);
        NumOfStuffedBits = NumOfStuffedBits + 1;
        stuffed_frame(i + NumOfStuffedBits) = 1;
        
    elseif NumOfOnes == 5
        NumOfOnes = 0;
        NumOfZeros = NumOfZeros + 1;
        
        %Appending the stuffed ZERO
        stuffed_frame(i + NumOfStuffedBits) = frame(i);
        NumOfStuffedBits = NumOfStuffedBits + 1;
        stuffed_frame(i + NumOfStuffedBits) = 0;
        
    else
        stuffed_frame(i + NumOfStuffedBits) = frame(i); 
    end
end
stuffed_frame_length = length(frame) + NumOfStuffedBits;
end

== matlab function CAN_Model_v5/CanNode1/Triggered Subsystem1/MATLAB Function ==
  data: Init input; InitCmplt output; Bus input; index input; next_index output
function [InitCmplt, next_index] = BusIdleSensing(Init, Bus, index)

InitCmplt = 0;

if Init == 1
    if Bus == 1
        if index < 10 %Number of one to wait for EOF (after 11 ones)
            next_index = index + 1;
        else
            next_index = 0;
            InitCmplt = 1;
        end
    else
        next_index = 0;
    end
else
   next_index = 0;
end

end

== matlab function CAN_Model_v5/CanNode1/Triggered Subsystem1/MATLAB Function1 ==
  data: Bus input; SOF output; BusIdle input
function SOF = SOF_Detection(Bus, BusIdle)

if BusIdle == 1 %Checks the current state of the FSM
    if Bus == 0
        SOF = 1; %SOF Detected, the flag goes to One!
    else
        SOF = 0;    
    end
else
    SOF = 0;
end

end

== matlab function CAN_Model_v5/CanNode1/Triggered Subsystem1/MATLAB Function2 ==
  data: ArbCmplt output; Win output; Arbitration input; Bus input; ID input; ID_Lenght input; next_index output; index input
function [ArbCmplt, Win, next_index] = arbitration(Arbitration, Bus, ID, ID_Lenght, index)

ArbCmplt = 0;
Win = 0;
next_index = 1;

if Arbitration == 1
    if index <= ID_Lenght
        if ID(index) == Bus
            next_index = index + 1;
        else
            Win = 0;
            ArbCmplt = 1;
        end
    else
        next_index = 1;
        Win = 1;
        ArbCmplt = 1;
    end    
    
else next_index = 1;
    
end
end

== matlab function CAN_Model_v5/Triggered Subsystem/MATLAB Function ==
  data: NodesID input; nextID output; TxCmplt input; RTS_Inc input; ID input; RTS input; Count input; nextRTS output; nextCount output
function [nextID, nextRTS, nextCount] = fcn(NodesID, TxCmplt, RTS_Inc, ID, RTS, Count)

NumOfNodes = size(NodesID);
temp = 0;

if Count < RTS_Inc
    nextCount = Count + 1;
else
    nextCount = 0;
    temp = temp + 1;
end

if TxCmplt == 1
    temp = temp - 1;
    nextID = NodesID( randi([1,NumOfNodes(1)]) ,:);
else
    nextID = ID';
end

nextRTS = RTS + temp;

end

== matlab function CAN_Model_v5/Triggered Subsystem1/MATLAB Function ==
  data: Timer input; nextRTS output; TxCmplt input; RTS input; Count input; nextCount output
function [nextRTS, nextCount] = fcn(Timer, TxCmplt, RTS, Count)
temp = 0;

if Count < Timer
    nextCount = Count + 1;
else
    nextCount = 0;
    temp = temp + 1;
end

if TxCmplt == 1
    temp = temp - 1;
end

nextRTS = RTS + temp;

end

== matlab function CAN_Model_v5/CanNode/Receiver/MATLAB BusRxAndDestuff ==
  data: Bus input; EOF output; ACK output; Enable input; AckEnable input; Frame input; Index input; Error output; DeStuffedFrame output; NextFrame output; NextIndex output; Count input; NextCount output; Jump input; NextJump output
function [EOF, ACK, Error, DeStuffedFrame, NextFrame, NextIndex, NextCount, NextJump] = BusRxAndDestuff(Bus, Enable, AckEnable, Frame, Index, Count, Jump)

DeStuffedFrame = zeros(110,1);
NextCount = 0;
NextFrame = zeros(110,1);
EOF = 0;
Error = 0;
NextIndex = 1;
NextJump = 0;
ACK = 1;

if Enable == 1
    if Index <= 110
        NextFrame = Frame;
        if (Index <= 98) || (Count == 4)
            if (Index == 1) || (Jump == 1)
                NextFrame(Index) = Bus;
                NextIndex = Index + 1;
            else
                if Count == 4
                    NextIndex = Index;
                    NextCount = 0;
                    NextJump = 1;
                else
                    NextFrame(Index) = Bus;
                    NextIndex = Index + 1;
                    if Bus == NextFrame(Index - 1)
                        NextCount = Count + 1;
                    else
                        NextCount = 0;
                    end
                end
            end
        else
            if(Index == 99) && (AckEnable == 1)
                ACK = 0;
            end
            NextFrame(Index) = Bus;
            NextIndex = Index + 1;
        end
    else
        EOF = 1;
        DeStuffedFrame = Frame;
    end
end
end
